simulink model "DriverModel_DynamicsSimple"  (Simulink 7.6)
settings: Solver=ode45  StartTime=0.0  StopTime=10.0  RelTol=1e-3
undefined symbols (not defined in the file): I0, Vinit
settings Model: Creator=pastora  LastModifiedBy=pastora
settings OptimizationCC: InitFltsAndDblsToZero=on
settings DebuggingCC: SaveWithParameterizedLinksMsg=none  SignalResolutionControl=TryResolveAllWithWarning  MultiTaskDSMMsg=warning  MultiTaskCondExecSysMsg=none  StrictBusMsg=Warning
settings RTWCC: IncludeERTFirstTime=on
settings GRTTargetCC: TargetFcnLib=ansi_tfl_tmw.mat

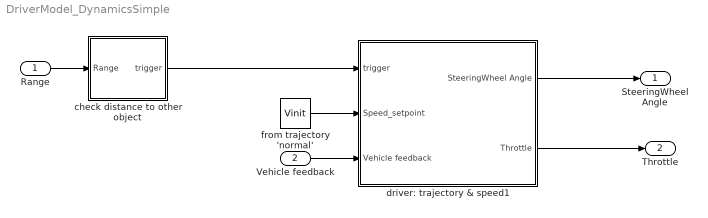
== system DriverModel_DynamicsSimple ==
  Range : Inport
  Vehicle feedback : Inport  Port=2
  check distance to other object : Subsystem
  driver: trajectory & speed1 : Subsystem
  from trajectory 'normal' : Constant  Value=Vinit
  SteeringWheel Angle : Outport
  Throttle : Outport  Port=2
  wires:
  check distance to other object/1(trigger) -> driver: trajectory & speed1/1(trigger)
  from trajectory 'normal'/1 -> driver: trajectory & speed1/2(Speed_setpoint)
  driver: trajectory & speed1/1(SteeringWheel Angle) -> SteeringWheel Angle/1
  driver: trajectory & speed1/2(Throttle) -> Throttle/1
  Vehicle feedback/1 -> driver: trajectory & speed1/3(Vehicle feedback)
  Range/1 -> check distance to other object/1(Range)

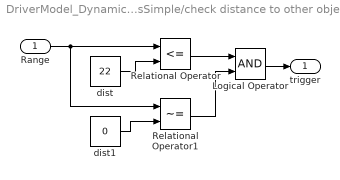
== system DriverModel_DynamicsSimple/check distance to other object ==
  Range : Inport
  Logical Operator : Logic  AllPortsSameDT=off  OutDataTypeStr=boolean
  Relational Operator : RelationalOperator  Operator=<=  OutDataTypeStr=boolean
  Relational Operator1 : RelationalOperator  Operator=~=  OutDataTypeStr=boolean
  dist : Constant  Value=22
  dist1 : Constant  Value=0
  trigger : Outport
  wires:
  Logical Operator/1 -> trigger/1
  Relational Operator1/1 -> Logical Operator/2
  Relational Operator/1 -> Logical Operator/1
  dist1/1 -> Relational Operator1/2
  dist/1 -> Relational Operator/2
  Range/1 -> Relational Operator/1, Relational Operator1/1

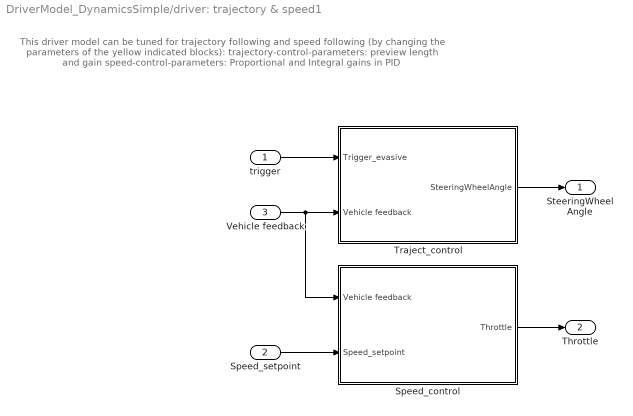
== system DriverModel_DynamicsSimple/driver: trajectory & speed1 ==
  note: This driver model can be tuned for trajectory following and speed following
      | (by changing the parameters of the yellow indicated blocks):
      |
      | trajectory-control-parameters: preview length and gain
      | speed-control-parameters: Proportional and Integral gains in PID
  trigger : Inport
  Speed_setpoint : Inport  Port=2
  Vehicle feedback : Inport  Port=3
  Speed_control : Subsystem
  Traject_control : Subsystem
  SteeringWheel Angle : Outport  InitialOutput=0
  Throttle : Outport  Port=2  InitialOutput=0
  wires:
  trigger/1 -> Traject_control/1(Trigger_evasive)
  Traject_control/1(SteeringWheelAngle) -> SteeringWheel Angle/1
  Vehicle feedback/1 -> Traject_control/2(Vehicle feedback), Speed_control/1(Vehicle feedback)
  Speed_control/1(Throttle) -> Throttle/1
  Speed_setpoint/1 -> Speed_control/2(Speed_setpoint)

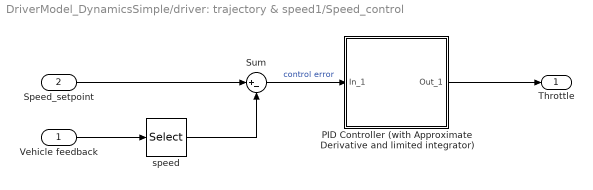
== system DriverModel_DynamicsSimple/driver: trajectory & speed1/Speed_control ==
  Vehicle feedback : Inport
  Speed_setpoint : Inport  Port=2
  PID Controller (with Approximate Derivative and limited integrator) : Subsystem  mask(PID(2) Controller){P=20, I=4, D=0, N=100}
      mask prompts: P "Proportional:"; I "Integral:"; D "Derivative:"; N "Derivative divisor(N):"
      mask help:
      | Enter Proportional(P), Integral(I), and Derivative(D) and divisor (N) terms.
      | P+I/s+Ds/(1/Ns+1)
      mask Help: This block implements a PID controller where parameters are entered for the Proportional, Integral and Derivative and divisor terms. Unmask this block to see how it works. The derivative term is implemented using an s/(s/N +1)  transfer function block. Making N large can create a "stiff" system.
      mask Display: disp('PID')
  Sum : Sum  Inputs=|+-
  speed : Selector  InputPortWidth=4  IndexOptions=Index vector (dialog)  Indices=4  OutputSizes=1
  Throttle : Outport
  wires:
  PID Controller (with Approximate Derivative and limited integrator)/1(Out_1) -> Throttle/1
  Vehicle feedback/1 -> speed/1
  Sum/1 -> PID Controller (with Approximate Derivative and limited integrator)/1(In_1)  "control error"
  speed/1 -> Sum/2
  Speed_setpoint/1 -> Sum/1

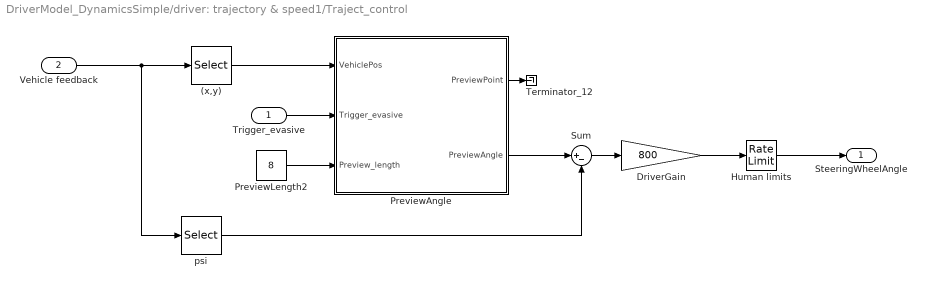
== system DriverModel_DynamicsSimple/driver: trajectory & speed1/Traject_control ==
  Trigger_evasive : Inport
  Vehicle feedback : Inport  Port=2
  (x,y) : Selector  InputPortWidth=4  IndexOptions=Index vector (dialog)  Indices=[1 2]  OutputSizes=1
  DriverGain : Gain  Gain=800
  Human limits : RateLimiter  RisingSlewLimit=360*2  FallingSlewLimit=-360*2  SampleTimeMode=inherited
  PreviewAngle : Subsystem  mask{FileName=normal_Synced.mat, FileName2=evasive.mat}
      mask prompts: FileName "Initial trajectory"; FileName2 "Evasive manoeuvre"
      mask init:
      | load(['trajectories/',FileName])
      | traject=trajectory';
      | 
      | load(['trajectories/',FileName2])
      | traject2 = trajectory';
  PreviewLength2 : Constant  Value=8
  Sum : Sum  Inputs=|+-
  Terminator_12 : Terminator
  psi : Selector  InputPortWidth=4  IndexOptions=Index vector (dialog)  Indices=3  OutputSizes=1
  SteeringWheelAngle : Outport  InitialOutput=0
  wires:
  (x,y)/1 -> PreviewAngle/1(VehiclePos)
  PreviewAngle/1(PreviewPoint) -> Terminator_12/1
  PreviewAngle/2(PreviewAngle) -> Sum/1
  psi/1 -> Sum/2
  Sum/1 -> DriverGain/1
  Vehicle feedback/1 -> (x,y)/1, psi/1
  DriverGain/1 -> Human limits/1
  Trigger_evasive/1 -> PreviewAngle/2(Trigger_evasive)
  PreviewLength2/1 -> PreviewAngle/3(Preview_length)
  Human limits/1 -> SteeringWheelAngle/1

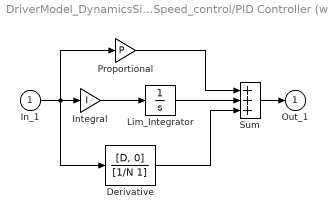
== system DriverModel_DynamicsSimple/driver: trajectory & speed1/Speed_control/PID Controller (with Approximate Derivative and limited integrator) ==
  In_1 : Inport
  Derivative : TransferFcn  Numerator=[D, 0]  Denominator=[1/N 1]
  Integral : Gain  Gain=I  SaturateOnIntegerOverflow=on  OutDataTypeStr=Inherit: Same as input  ParamDataTypeStr=Inherit: Same as input
  Lim_Integrator : Integrator  InitialCondition=I0  LimitOutput=on  LowerSaturationLimit=-0.1
  Proportional : Gain  Gain=P  SaturateOnIntegerOverflow=on  OutDataTypeStr=Inherit: Same as input  ParamDataTypeStr=Inherit: Same as input
  Sum : Sum  Inputs=+++  SaturateOnIntegerOverflow=on  InputSameDT=on  OutDataTypeStr=Inherit: Same as first input
  Out_1 : Outport  InitialOutput=0
  wires:
  Sum/1 -> Out_1/1
  In_1/1 -> Derivative/1, Proportional/1, Integral/1
  Derivative/1 -> Sum/3
  Lim_Integrator/1 -> Sum/2
  Proportional/1 -> Sum/1
  Integral/1 -> Lim_Integrator/1

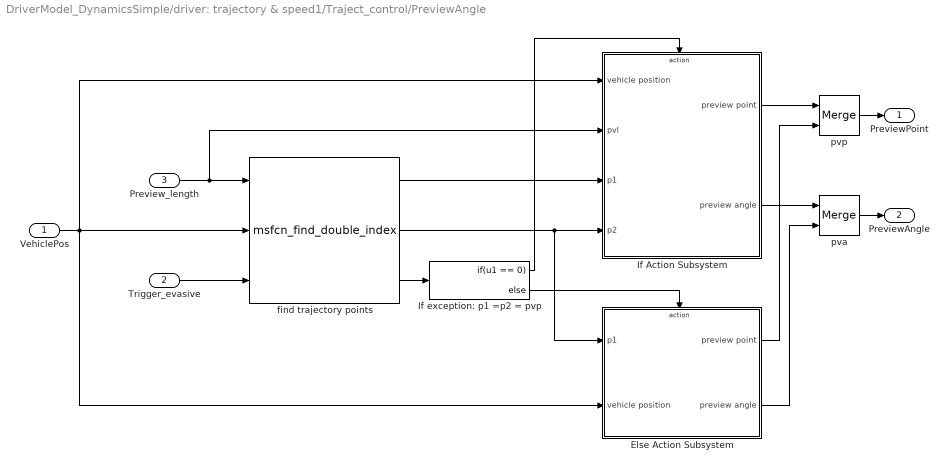
== system DriverModel_DynamicsSimple/driver: trajectory & speed1/Traject_control/PreviewAngle ==
  VehiclePos : Inport
  Trigger_evasive : Inport  Port=2
  Preview_length : Inport  Port=3
  Else Action Subsystem : Subsystem  TreatAsAtomicUnit=on
  If Action Subsystem : Subsystem  TreatAsAtomicUnit=on
  If exception: p1 =p2 = pvp : If  IfExpression=u1 == 0
  find trajectory points : M-S-Function  FunctionName=msfcn_find_double_index  Parameters=[traject(:,2) traject(:,3)], [traject2(:,2) traject2(:,3)]
  pva : Merge  InitialOutput=0
  pvp : Merge  InitialOutput=[0 0]
  PreviewPoint : Outport
  PreviewAngle : Outport  Port=2
  wires:
  VehiclePos/1 -> find trajectory points/2, Else Action Subsystem/2(vehicle position), If Action Subsystem/1(vehicle position)
  find trajectory points/3 -> If exception: p1 =p2 = pvp/1
  find trajectory points/1 -> If Action Subsystem/3(p1)
  find trajectory points/2 -> If Action Subsystem/4(p2), Else Action Subsystem/1(p1)
  If exception: p1 =p2 = pvp/1 -> If Action Subsystem/Action
  If Action Subsystem/1(preview point) -> pvp/1
  Else Action Subsystem/1(preview point) -> pvp/2
  If Action Subsystem/2(preview angle) -> pva/1
  Else Action Subsystem/2(preview angle) -> pva/2
  If exception: p1 =p2 = pvp/2 -> Else Action Subsystem/Action
  pvp/1 -> PreviewPoint/1
  pva/1 -> PreviewAngle/1
  Trigger_evasive/1 -> find trajectory points/3
  Preview_length/1 -> find trajectory points/1, If Action Subsystem/2(pvl)

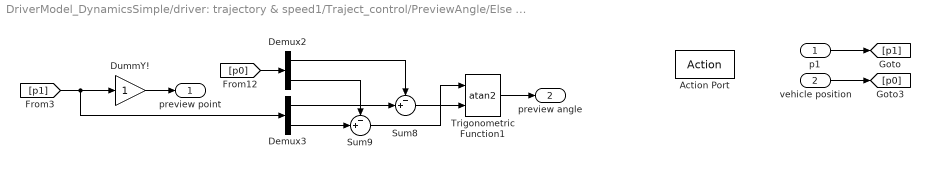
== system DriverModel_DynamicsSimple/driver: trajectory & speed1/Traject_control/PreviewAngle/Else Action Subsystem ==
  p1 : Inport
  vehicle position : Inport  Port=2
  Action Port : ActionPort  InitializeStates=reset
  Demux2 : Demux  Outputs=2
  Demux3 : Demux  Outputs=2
  DummY! : Gain
  Sum8 : Sum  Inputs=-+|
  Sum9 : Sum  Inputs=-+|
  Trigonometric Function1 : Trigonometry  Operator=atan2
  preview point : Outport
  preview angle : Outport  Port=2
  wires:
  Sum8/1 -> Trigonometric Function1/2
  Sum9/1 -> Trigonometric Function1/1
  [p0] -> Demux2/1
  Trigonometric Function1/1 -> preview angle/1
  Demux3/2 -> Sum9/2
  Demux2/2 -> Sum9/1
  Demux2/1 -> Sum8/1
  Demux3/1 -> Sum8/2
  [p1] -> Demux3/1, DummY!/1
  p1/1 -> [p1]
  vehicle position/1 -> [p0]
  DummY!/1 -> preview point/1

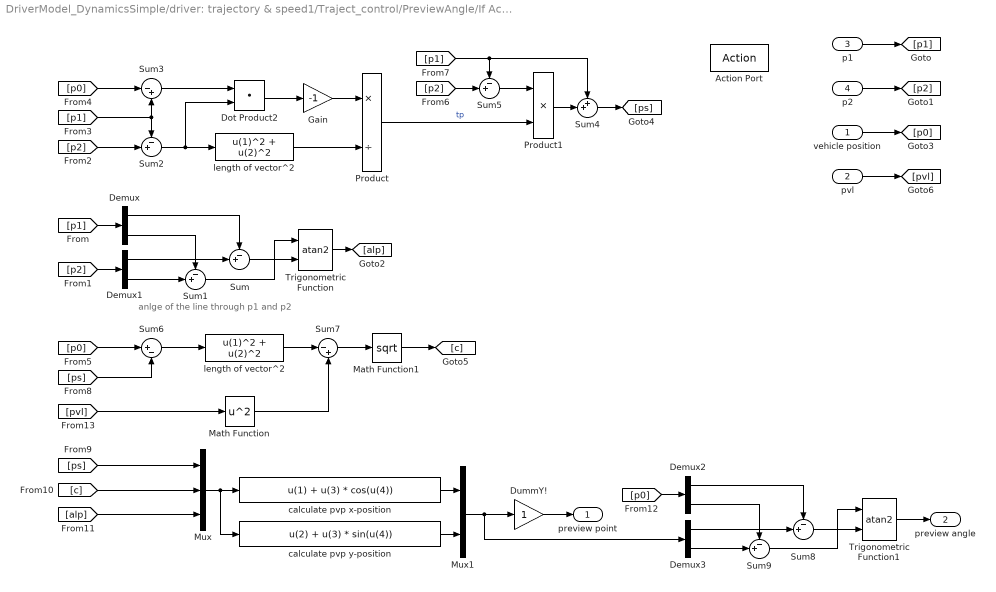
== system DriverModel_DynamicsSimple/driver: trajectory & speed1/Traject_control/PreviewAngle/If Action Subsystem ==
  note: anlge of the line through p1 and p2
  vehicle position : Inport
  pvl : Inport  Port=2
  p1 : Inport  Port=3
  p2 : Inport  Port=4
  Action Port : ActionPort  InitializeStates=reset
  Demux{,1..3} (4 alike) : Demux  Outputs=2
  Dot Product2 : DotProduct  InputSameDT=on  OutDataTypeStr=Inherit: Inherit via internal rule
  DummY! : Gain
  Gain : Gain  Gain=-1
  Math Function : Math  Operator=square  SaturateOnIntegerOverflow=on
  Math Function1 : Math  Operator=sqrt  SaturateOnIntegerOverflow=on
  Mux : Mux  Inputs=3
  Mux1 : Mux  Inputs=2
  Product : Product  Inputs=*/  RndMeth=Zero
  Product1 : Product  RndMeth=Zero
  Sum{,1..2,5,8..9} (6 alike) : Sum  Inputs=-+|
  Sum3 : Sum  Inputs=|-+
  Sum4 : Sum  Inputs=++|
  Sum6 : Sum  Inputs=|+-
  Sum7 : Sum  Inputs=|-+
  Trigonometric Function : Trigonometry  Operator=atan2
  Trigonometric Function1 : Trigonometry  Operator=atan2
  calculate pvp x-position : Fcn  Expr=u(1) + u(3) * cos(u(4))
  calculate pvp y-position : Fcn  Expr=u(2) + u(3) * sin(u(4))
  length of vector^2 : Fcn  Expr=u(1)^2 + u(2)^2
  "length of vector^2 " : Fcn  Expr=u(1)^2 + u(2)^2
  preview point : Outport
  preview angle : Outport  Port=2
  wires:
  vehicle position/1 -> [p0]
  Demux1/1 -> Sum/2
  Demux/1 -> Sum/1
  Demux/2 -> Sum1/1
  Demux1/2 -> Sum1/2
  Trigonometric Function/1 -> [alp]
  p1/1 -> [p1]
  p2/1 -> [p2]
  [p1] -> Demux/1
  [p2] -> Demux1/1
  [p2] -> Sum2/2
  [p1] -> Sum2/1, Sum3/2
  Sum2/1 -> length of vector^2/1, Dot Product2/2
  [p0] -> Sum3/1
  Sum3/1 -> Dot Product2/1
  Dot Product2/1 -> Gain/1
  Gain/1 -> Product/1
  length of vector^2/1 -> Product/2
  Product/1 -> Product1/2  "tp"
  [p2] -> Sum5/2
  [p1] -> Sum5/1, Sum4/1
  Sum5/1 -> Product1/1
  Product1/1 -> Sum4/2
  Sum4/1 -> [ps]
  [p0] -> Sum6/1
  [ps] -> Sum6/2
  Sum6/1 -> "length of vector^2 "/1
  "length of vector^2 "/1 -> Sum7/1
  [pvl] -> Math Function/1
  Math Function/1 -> Sum7/2
  Sum7/1 -> Math Function1/1
  Math Function1/1 -> [c]
  [ps] -> Mux/1
  [c] -> Mux/2
  [alp] -> Mux/3
  Mux/1 -> calculate pvp x-position/1, calculate pvp y-position/1
  calculate pvp x-position/1 -> Mux1/1
  calculate pvp y-position/1 -> Mux1/2
  Mux1/1 -> Demux3/1, DummY!/1
  Sum1/1 -> Trigonometric Function/1
  Sum/1 -> Trigonometric Function/2
  Demux3/1 -> Sum8/2
  Demux2/1 -> Sum8/1
  Demux2/2 -> Sum9/1
  Demux3/2 -> Sum9/2
  Trigonometric Function1/1 -> preview angle/1
  [p0] -> Demux2/1
  Sum9/1 -> Trigonometric Function1/1
  Sum8/1 -> Trigonometric Function1/2
  DummY!/1 -> preview point/1
  pvl/1 -> [pvl]
